simulink model "SelfBalancingEV_V1"  (R2022a)
settings: Solver=VariableStepAuto  StartTime=0.0  StopTime=10.0  RelTol=1e-3
InitFcn:
  | m = 100
  | g = 9.81
  | I = 5
  | R = 2
  | v0 =100
undefined symbols (not defined in the file): Ion, Lithium, sigbuilder_block
libraries: simulink x4, powerlib x2, slpidlib x1, electricdrivelib x1
settings Model: Creator=DELL  LastModifiedBy=DELL

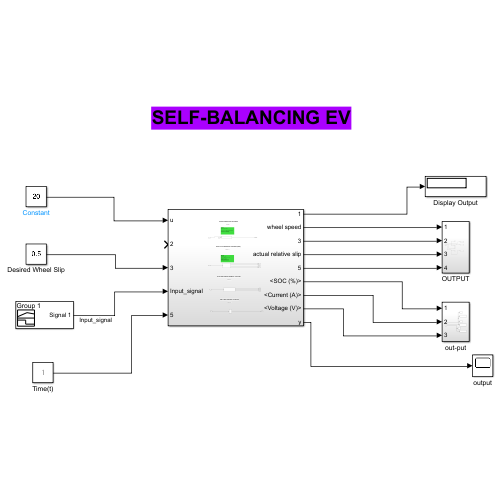
[thumbnail: Simulink's stored preview of the top-level diagram]
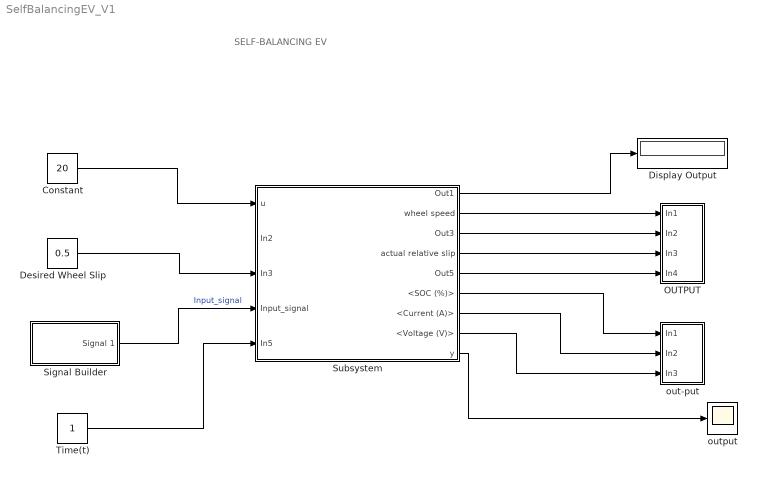
== system SelfBalancingEV_V1 ==
  note: SELF-BALANCING EV
  Constant : Constant  Value=20
  Desired Wheel Slip : Constant  Value=0.5
  Display Output : Display
  OUTPUT : Subsystem
  Signal Builder : Subsystem  Tag=STV Subsys  LoadFcn=sigbuilder_block('load');  StartFcn=sigbuilder_block('start');  StopFcn=sigbuilder_block('stop');  ClipboardFcn=sigbuilder_block('clipboard');  mask(Sigbuilder block){tuvar=[0:10]}
      mask help: Simulink:masks:SigbuilderBlock_MD
      mask init:
      | if ~strcmp(get_param(bdroot(gcbh),'SimulationStatus'),'stopped') tuvar = sigbuilder_block('maskInit'); end
      settings: CopyFcn=sigbuilder_block('copy');  DeleteFcn=sigbuilder_block('delete');  ModelCloseFcn=sigbuilder_block('modelClose');  PreSaveFcn=sigbuilder_block('preSave');  PauseFcn=sigbuilder_block('pause');  ContinueFcn=sigbuilder_block('continue');  NameChangeFcn=sigbuilder_block('namechange');  OpenFcn=sigbuilder_block('open',[406.8 120.6 550.8 400.2 ]);  CloseFcn=sigbuilder_block('close');
      mask Display: plot(0, 0, 100, 100,[2, 2, 32, 32, 2], [68, 8, 8, 68, 68],[32, 2], [38, 38], [32, 19, 2],[53, 60, 44], [32, 17, 17, 2],[16, 16, 31, 31]);txt = getActiveGroup(gcbh);text(2, 100, txt,'verticalAlignment', 'top');
  Subsystem : Subsystem
  Time(t) : Constant
  out-put : Subsystem
  output : Scope
  wires:
  Constant/1 -> Subsystem/1(u)
  Desired Wheel Slip/1 -> Subsystem/3(In3)
  Signal Builder/1(Signal 1) -> Subsystem/4(Input_signal)  "Input_signal"
  Time(t)/1 -> Subsystem/5(In5)
  Subsystem/1(Out1) -> Display Output/1
  Subsystem/2(wheel speed) -> OUTPUT/1(In1)
  Subsystem/3(Out3) -> OUTPUT/2(In2)
  Subsystem/4(actual relative slip) -> OUTPUT/3(In3)
  Subsystem/5(Out5) -> OUTPUT/4(In4)
  Subsystem/6(<SOC (%)>) -> out-put/1(In1)
  Subsystem/7(<Current (A)>) -> out-put/2(In2)
  Subsystem/8(<Voltage (V)>) -> out-put/3(In3)
  Subsystem/9(y) -> output/1

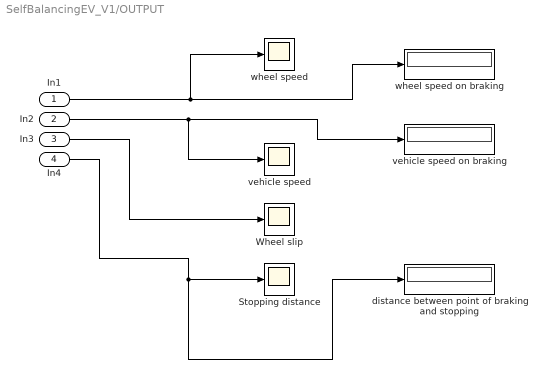
== system SelfBalancingEV_V1/OUTPUT ==
  In1 : Inport
  In2 : Inport  Port=2
  In3 : Inport  Port=3
  In4 : Inport  Port=4
  Stopping distance : Scope
  Wheel slip : Scope
  distance between point of braking and stopping : Display
  vehicle speed : Scope
  vehicle speed on braking : Display
  wheel speed : Scope
  wheel speed on braking : Display
  wires:
  In1/1 -> wheel speed on braking/1, wheel speed/1
  In4/1 -> distance between point of braking and stopping/1, Stopping distance/1
  In2/1 -> vehicle speed/1, vehicle speed on braking/1
  In3/1 -> Wheel slip/1

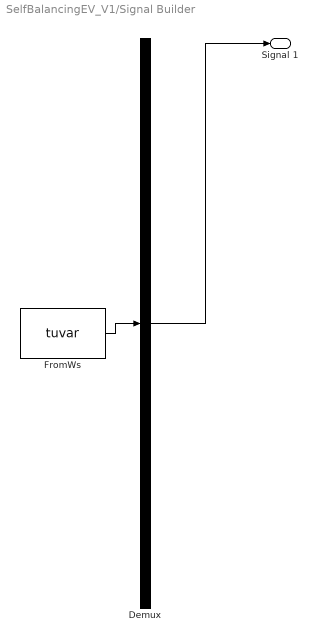
== system SelfBalancingEV_V1/Signal Builder ==
  Demux : Demux  Tag=STV Demux  Outputs=1
      settings: DisplayOption=none
  FromWs : FromWorkspace  Tag=STV FromWs  VariableName=tuvar
      SigBuilderData=|
      | common.afterFinalStr = 'Extrapolate'
      | common.sampleTime = 0
      | dataSet.timeRange = [0 10]
      | dataSet.name = 'Group 1'
      | sbobj.Groups.Name = 'Group 1'
      | sbobj.Groups.Signals.Name = 'Signal 1'
      | sbobj.Groups.Signals.XData = [0 1.94 2.9 4 4 4.88 5.98 6.66 6.66 7.76 10]
      | sbobj.Groups.Signals.YData = [0 0.345 0.345 0 0.435 0.875 0.99435 1 0 0.275 0]
  Signal 1 : Outport  Tag=STV Outport
  wires:
  Demux/1 -> Signal 1/1
  FromWs/1 -> Demux/1

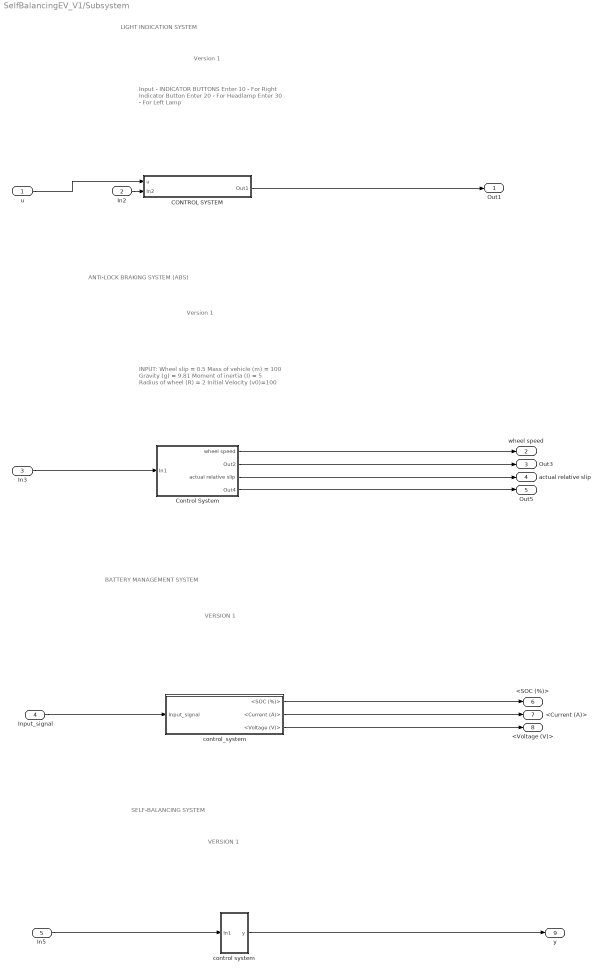
== system SelfBalancingEV_V1/Subsystem ==
  note: VERSION 1
  note: BATTERY MANAGEMENT SYSTEM
  note: VERSION 1
  note: SELF-BALANCING SYSTEM
  note: LIGHT INDICATION SYSTEM
  note: Input -
      | INDICATOR BUTTONS
      |
      | Enter 10 - For Right Indicator Button
      | Enter 20 - For Headlamp
      | Enter 30 - For Left Lamp
  note: Version 1
  note: Version 1
  note: INPUT:
      | Wheel slip = 0.5
      | Mass of vehicle (m) = 100
      | Gravity (g) = 9.81
      | Moment of inertia (I) = 5
      | Radius of wheel (R) = 2
      | Initial Velocity (v0)=100
  note: ANTI-LOCK BRAKING SYSTEM (ABS)
  u : Inport
  In2 : Inport  Port=2
  In3 : Inport  Port=3
  Input_signal : Inport  Port=4
  In5 : Inport  Port=5
  CONTROL SYSTEM : Subsystem
  Control System : Subsystem
  control system : Subsystem
  control_system : Subsystem
  Out1 : Outport
  wheel speed : Outport  Port=2
  Out3 : Outport  Port=3
  actual relative slip : Outport  Port=4
  Out5 : Outport  Port=5
  <SOC (%)> : Outport  Port=6
  <Current (A)> : Outport  Port=7
  <Voltage (V)> : Outport  Port=8
  y : Outport  Port=9
  wires:
  CONTROL SYSTEM/1(Out1) -> Out1/1
  In3/1 -> Control System/1(In1)
  control system/1(y) -> y/1
  u/1 -> CONTROL SYSTEM/1(u)
  control_system/1(<SOC (%)>) -> <SOC (%)>/1
  Control System/2(Out2) -> Out3/1
  control_system/2(<Current (A)>) -> <Current (A)>/1
  Control System/3(actual relative slip) -> actual relative slip/1
  In5/1 -> control system/1(In1)
  control_system/3(<Voltage (V)>) -> <Voltage (V)>/1
  In2/1 -> CONTROL SYSTEM/2(In2)
  Input_signal/1 -> control_system/1(Input_signal)
  Control System/1(wheel speed) -> wheel speed/1
  Control System/4(Out4) -> Out5/1

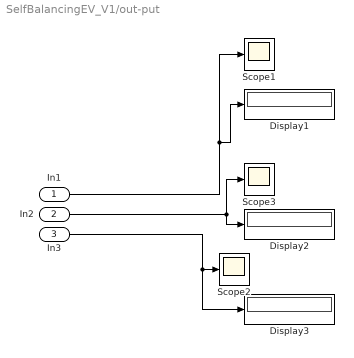
== system SelfBalancingEV_V1/out-put ==
  In1 : Inport
  In2 : Inport  Port=2
  In3 : Inport  Port=3
  Display1 : Display
  Display2 : Display
  Display3 : Display
  Scope1 : Scope
  Scope2 : Scope
  Scope3 : Scope
  wires:
  In1/1 -> Scope1/1, Display1/1
  In3/1 -> Display3/1, Scope2/1
  In2/1 -> Scope3/1, Display2/1

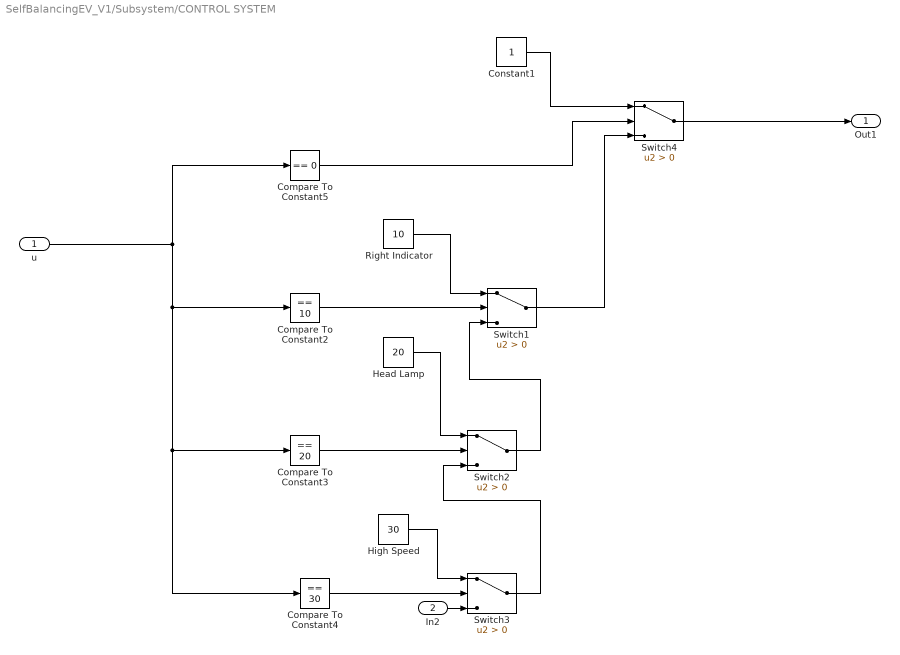
== system SelfBalancingEV_V1/Subsystem/CONTROL SYSTEM ==
  u : Inport
  In2 : Inport  Port=2
  Compare To Constant2 : simulink/Logic and Bit Operations/Compare To Constant  relop===  const=10  OutDataTypeStr=boolean
  Compare To Constant3 : simulink/Logic and Bit Operations/Compare To Constant  relop===  const=20  OutDataTypeStr=boolean
  Compare To Constant4 : simulink/Logic and Bit Operations/Compare To Constant  relop===  const=30  OutDataTypeStr=boolean
  Compare To Constant5 : simulink/Logic and Bit Operations/Compare To Constant  relop===  const=0  OutDataTypeStr=boolean
  Constant1 : Constant
  Head Lamp : Constant  Value=20
  High Speed : Constant  Value=30
  Right Indicator : Constant  Value=10
  Switch{1..4} (4 alike) : Switch  Criteria=u2 > Threshold  SaturateOnIntegerOverflow=off  InputSameDT=off
  Out1 : Outport
  wires:
  Compare To Constant2/1 -> Switch1/2
  Switch2/1 -> Switch1/3
  u/1 -> Compare To Constant4/1, Compare To Constant3/1, Compare To Constant2/1, Compare To Constant5/1
  Switch1/1 -> Switch4/3
  Compare To Constant5/1 -> Switch4/2
  Head Lamp/1 -> Switch2/1
  Compare To Constant4/1 -> Switch3/2
  Switch3/1 -> Switch2/3
  Right Indicator/1 -> Switch1/1
  High Speed/1 -> Switch3/1
  Compare To Constant3/1 -> Switch2/2
  Constant1/1 -> Switch4/1
  Switch4/1 -> Out1/1
  In2/1 -> Switch3/3

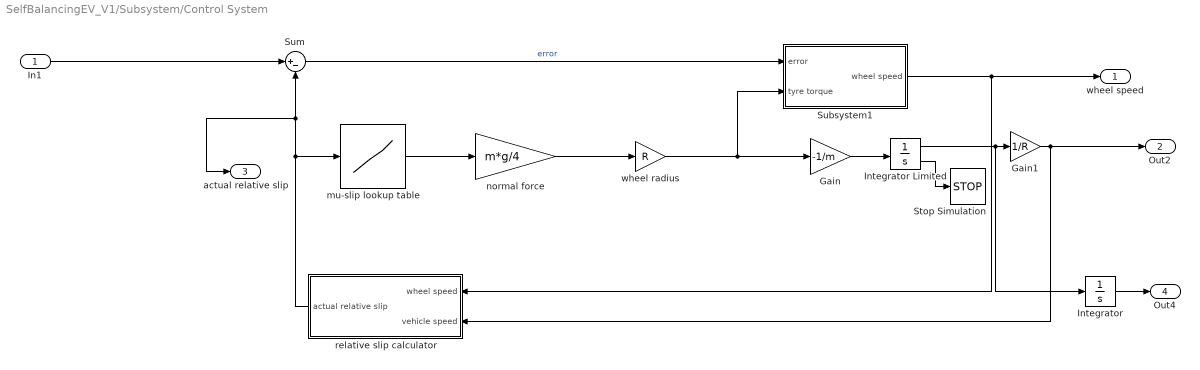
== system SelfBalancingEV_V1/Subsystem/Control System ==
  In1 : Inport
  Gain : Gain  Gain=-1/m
  Gain1 : Gain  Gain=1/R
  Integrator : Integrator
  Integrator Limited : Integrator  InitialCondition=v0  LimitOutput=on  UpperSaturationLimit=1000  LowerSaturationLimit=0  ShowSaturationPort=on
  Stop Simulation : Stop
  Subsystem1 : Subsystem
  Sum : Sum  Inputs=|+-
  mu-slip lookup table : Lookup_n-D  NumberOfTableDimensions=1  BreakpointsForDimension1=[0;0.05;0.1;0.15;0.2;0.25;0.3;0.35;0.4;0.45;0.5;0.55;0.6;0.65;0.7;0.75;0.8;0.85;0.9;0.95;1]  Table=[0;0.4;0.8;0.97;1;0.98;0.96;0.94;0.92;0.9;0.88;0.855;0.83;0.81;0.79;0.77;0.75;0.73;0.72;0.71;0.7]  InternalRulePriority=Speed  RndMeth=Simplest
  normal force : Gain  Gain=m*g/4
  relative slip calculator : Subsystem
  wheel radius : Gain  Gain=R
  wheel speed : Outport
  Out2 : Outport  Port=2
  actual relative slip : Outport  Port=3
  Out4 : Outport  Port=4
  wires:
  Gain/1 -> Integrator Limited/1
  normal force/1 -> wheel radius/1
  wheel radius/1 -> Gain/1, Subsystem1/2(tyre torque)
  Integrator Limited/1 -> Integrator/1, Gain1/1
  In1/1 -> Sum/1
  Subsystem1/1(wheel speed) -> wheel speed/1, relative slip calculator/1(wheel speed)
  Integrator Limited/2 -> Stop Simulation/1
  Sum/1 -> Subsystem1/1(error)  "error"
  relative slip calculator/1(actual relative slip) -> mu-slip lookup table/1, Sum/2, actual relative slip/1
  mu-slip lookup table/1 -> normal force/1
  Gain1/1 -> Out2/1, relative slip calculator/2(vehicle speed)
  Integrator/1 -> Out4/1

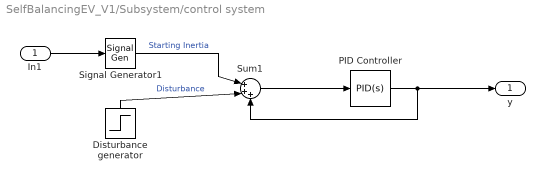
== system SelfBalancingEV_V1/Subsystem/control system ==
  In1 : Inport
  "Disturbance generator " : Step  Time=0.01  Before=010  After=10  SampleTime=0
  PID Controller : slpidlib/PID Controller  Controller=PID  Form=Parallel  TimeDomain=Continuous-time  UseExternalTs=off  SampleTime=-1  IntegratorMethod=Forward Euler  FilterMethod=Forward Euler  ControllerParametersSource=internal  P=1  I=1  UseKiTs=off  D=0  N=100  UseFilter=on  TunerSelectOption=Transfer Function Based (PID Tuner App)  InitialConditionSource=internal  InitialConditionForIntegrator=0  InitialConditionForFilter=0  DifferentiatorICPrevScaledInput=0  ExternalReset=none  TrackingMode=off  Kt=1  LimitOutput=off  SatLimitsSource=internal  UpperSaturationLimit=inf  LowerSaturationLimit=-inf  LinearizeAsGain=on  AntiWindupMode=none  Kb=1  POutMin=[]  POutMax=[]  IOutMin=[]  IOutMax=[]  DOutMin=[]  DOutMax=[]  NOutMin=[]  NOutMax=[]  SumOutMin=[]  SumOutMax=[]  SaturationOutMin=[]  SaturationOutMax=[]  PParamMin=[]  PParamMax=[]  IParamMin=[]  IParamMax=[]  DParamMin=[]  DParamMax=[]  NParamMin=[]  NParamMax=[]  KbParamMin=[]  KbParamMax=[]  KtParamMin=[]  KtParamMax=[]  KbOutMin=[]  KbOutMax=[]  KtOutMin=[]  KtOutMax=[]  IntegratorOutMin=[]  IntegratorOutMax=[]  FilterOutMin=[]  FilterOutMax=[]  SumI1OutMin=[]  SumI1OutMax=[]  SumI2OutMin=[]  SumI2OutMax=[]  SumI3OutMin=[]  SumI3OutMax=[]  SumI4OutMin=[]  SumI4OutMax=[]  SumDOutMin=[]  SumDOutMax=[]  DifferentiatorOutMin=[]  DifferentiatorOutMax=[]  FilterDiffOutCoefMin=[]  FilterDiffOutCoefMax=[]  ReciprocalOutMin=[]  ReciprocalOutMax=[]  SumDenOutMin=[]  SumDenOutMax=[]  SumNumOutMin=[]  SumNumOutMax=[]  DivideOutMin=[]  DivideOutMax=[]  UdiffTsProdOutMin=[]  UdiffTsProdOutMax=[]  NTsProdOutMin=[]  NTsProdOutMax=[]  UintegralTsProdOutMin=[]  UintegralTsProdOutMax=[]  UngainTsProdOutMin=[]  UngainTsProdOutMax=[]  IntegratorContinuousStateAttributes=''  IntegratorStateMustResolveToSignalObject=off  IntegratorRTWStateStorageClass=Auto  FilterContinuousStateAttributes=''  FilterStateMustResolveToSignalObject=off  FilterRTWStateStorageClass=Auto  ParallelPVariant=InternalParameters  IdealPVariant=Disabled  IVariant=InternalParameters  DVariant=InternalParameters  IntegratorVariant=Continuous  SatVariant=Disabled  AWVariant=Passthrough  PCopyVariant=Disabled  TRVariant=Disabled  FdbkBlocksVariant=Forward  IdealPFdbkVariant=Disabled  SatFdbkVariant=Disabled  DerivativeFilterVariant=ContFilter  NVariant=InternalParameters  NCopyVariant=Disabled  FilterICVariant=InternalICsFilter  IntegratorICVariant=InternalICs  ExternalResetVariant=Disabled  TRSumVariant=Passthrough  SumFdbkVariant=Disabled  SumVariant=Sum_PID  TsampFilterVariant=InternalTs  TsampNgainVariant=Passthrough  TsampIntegralVariant=Passthrough  ExternalSaturationOutDataTypeStr=Inherit: Same as second input  aMode=0
  Signal Generator1 : SignalGenerator  TimeSource=Use external signal  Frequency=2
  Sum1 : Sum  Inputs=|+++
  y : Outport
  wires:
  PID Controller/1 -> y/1, Sum1/3
  In1/1 -> Signal Generator1/1
  "Disturbance generator "/1 -> Sum1/2  "Disturbance"
  Signal Generator1/1 -> Sum1/1  "Starting Inertia"
  Sum1/1 -> PID Controller/1

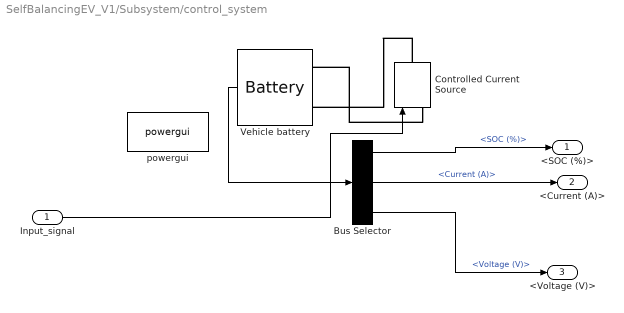
== system SelfBalancingEV_V1/Subsystem/control_system ==
  Input_signal : Inport
  Bus Selector : BusSelector  OutputSignals=SOC (%),Current (A),Voltage (V)
  Controlled Current Source : powerlib/Electrical Sources/Controlled Current Source  Initialize=on  Source_Type=AC  Amplitude=0  Phase=0  Frequency=0  Measurements=None
  Vehicle battery : electricdrivelib/Extra Sources/Battery  BatType=Lithium-Ion  ShowTempParam=off  ThermalPreset=no  ShowAgeParam=off  NomV=50  NomQ=50  SOC=100  Batt_Tr=30  PresetModel=on  MaxQ=50  MinV=37.5  FullV=58.1994  Dis_rate=21.7391  R=0.01  Normal_OP=45.2174  expZone="[54.0193      2.45652]"  current=[6.5 13 32.5]  Units=Time  Tci=20  NomT=20  T2=-30  MaxQ2=4.8  FullV2=7.1  Normal_OP2=5.655  expZone2="[6.58           1]"  Rca=0.6  ti=2000  Dp=0  Neq0=0  Tsim=1e6  Ta1=25  Qeol=5.4*0.9  Reol=0.013333*1.2  Char_age=[2.3478, 3]  Dis_age=[2.3478, 10]  N1=1500  N2=10500  N3=1000  N4=1400  Ta2=45  N5=950
  powergui : powerlib/powergui  Priority=1  SimulationMode=Continuous  SampleTime=50e-6  frequency=60  Iterations=50  frequencyindice=0  Pbase=100e6  ErrMax=1e-4  UnitsV=kV  UnitsW=MW  buscounter=0  FunctionMessages=off  echomessages=off  EnableUseOfTLC=off  CurrentSourceSwitches=off  DisableSnubberDevices=off  DisableRonSwitches=off  DisableVfSwitches=off  DisplayEquations=off  AutomaticDiscreteSolvers=off  SolverType=Tustin/Backward Euler (TBE)  Interpol=off  ExternalGateDelay=off  methode=off  Ts=100  x0status=blocks  SPID=on  SwTol=0  HookPort=off  NonlinearTolerance=1e-4  nMaxIteration=100  ContinueOnMaxIteration=off  RestoreLinks=warning  ResistiveCurrentMeasurement=off  Frange=[0:2:500]  Ylog=off  Xlog=on  ShowGrid=off  save=off  variable=ZData  structure=0  ZoomFFT=off  StartTime=0.0  cycles=1  DisplayStyle=1  fundamental=60  FreqAxis=off  MaxFrequency=1000  frequencyindicesteady=1  RmsSteady=1  display=off
  <SOC (%)> : Outport
  <Current (A)> : Outport  Port=2
  <Voltage (V)> : Outport  Port=3
  wires:
  Bus Selector/1 -> <SOC (%)>/1  "<SOC (%)>"
  Bus Selector/2 -> <Current (A)>/1  "<Current (A)>"
  Vehicle battery/1 -> Bus Selector/1
  Bus Selector/3 -> <Voltage (V)>/1  "<Voltage (V)>"
  Input_signal/1 -> Controlled Current Source/1
  connections:
  Controlled Current Source/RConn1 -- Vehicle battery/LConn2
  Controlled Current Source/LConn1 -- Vehicle battery/LConn1

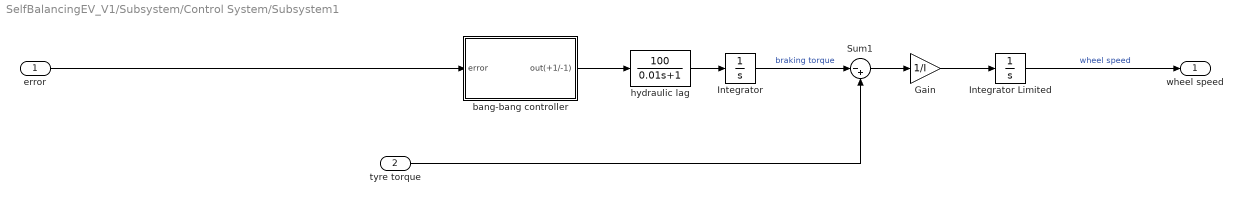
== system SelfBalancingEV_V1/Subsystem/Control System/Subsystem1 ==
  error : Inport
  tyre torque : Inport  Port=2
  Gain : Gain  Gain=1/I
  Integrator : Integrator  LimitOutput=on  UpperSaturationLimit=1000  LowerSaturationLimit=0
  Integrator Limited : Integrator  InitialCondition=v0/R  LimitOutput=on  UpperSaturationLimit=1000  LowerSaturationLimit=0
  Sum1 : Sum  Inputs=|-+
  bang-bang controller : Subsystem
  hydraulic lag : TransferFcn  Numerator=[100]  Denominator=[0.01 1]
  wheel speed : Outport
  wires:
  bang-bang controller/1(out(+1/-1)) -> hydraulic lag/1
  hydraulic lag/1 -> Integrator/1
  Integrator Limited/1 -> wheel speed/1  "wheel speed"
  Sum1/1 -> Gain/1
  error/1 -> bang-bang controller/1(error)
  Integrator/1 -> Sum1/1  "braking torque"
  Gain/1 -> Integrator Limited/1
  tyre torque/1 -> Sum1/2

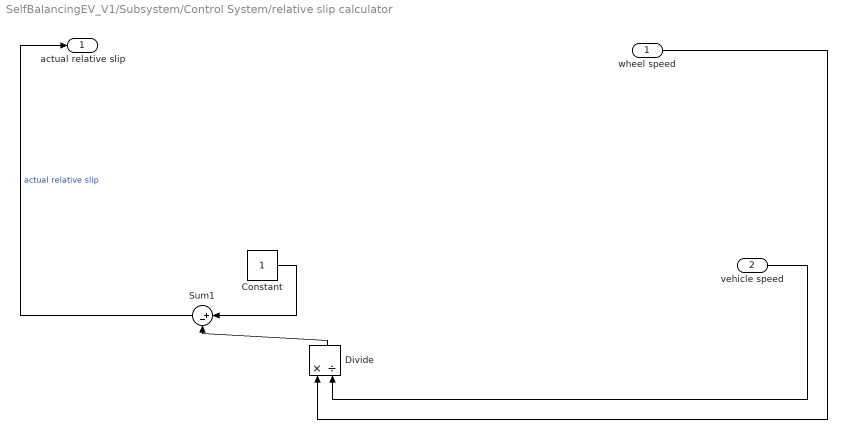
== system SelfBalancingEV_V1/Subsystem/Control System/relative slip calculator ==
  wheel speed : Inport
  vehicle speed : Inport  Port=2
  Constant : Constant
  Divide : Product  Inputs=*/
  Sum1 : Sum  Inputs=|+-
  actual relative slip : Outport
  wires:
  Divide/1 -> Sum1/2
  vehicle speed/1 -> Divide/2
  wheel speed/1 -> Divide/1
  Sum1/1 -> actual relative slip/1  "actual relative slip"
  Constant/1 -> Sum1/1

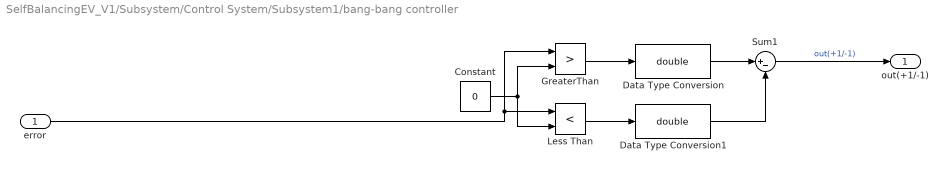
== system SelfBalancingEV_V1/Subsystem/Control System/Subsystem1/bang-bang controller ==
  error : Inport
  Constant : Constant  Value=0
  Data Type Conversion : DataTypeConversion  OutDataTypeStr=double  SaturateOnIntegerOverflow=off
  Data Type Conversion1 : DataTypeConversion  OutDataTypeStr=double  SaturateOnIntegerOverflow=off
  GreaterThan : RelationalOperator  Operator=>  OutDataTypeStr=boolean  RndMeth=Simplest  InputSameDT=off
  Less Than : RelationalOperator  Operator=<  OutDataTypeStr=boolean  RndMeth=Simplest  InputSameDT=off
  Sum1 : Sum  Inputs=|+-
  out(+1/-1) : Outport
  wires:
  Constant/1 -> Less Than/2, GreaterThan/2
  Data Type Conversion/1 -> Sum1/1
  GreaterThan/1 -> Data Type Conversion/1
  Less Than/1 -> Data Type Conversion1/1
  error/1 -> GreaterThan/1, Less Than/1
  Data Type Conversion1/1 -> Sum1/2
  Sum1/1 -> out(+1/-1)/1  "out(+1/-1)"
